simulink model "LeuchtenBox"  (R2017b)
settings: Solver=FixedStepAuto  StartTime=0.0  StopTime=10.0  RelTol=1e-3
PreLoadFcn:
  | waijung.modelPreload; % Required for working with Waijung Blockset. Do not remove.
undefined symbols (not defined in the file): HSEOSC, Link, LQFP100, m, n, ST, STM32F407VG
libraries: simulink x36, stm32f4_canbus_lib x10, stm32f4_io_lib x8, quarc_library x1, stm32f4_device_config_lib x1
CloseFcn:
  | waijung.modelClose; % Required for working with Waijung Blockset. Do not remove.
settings Model: Creator=labuser  LastModifiedBy=marti
settings OptimizationCC: DefaultParameterBehavior=Inlined  PassReuseOutputArgsAs=Individual arguments
settings DebuggingCC: ParameterTunabilityLossMsg=error
settings HardwareCC: ProdBitPerPointer=32  ProdBitPerSizeT=32  ProdBitPerPtrDiffT=32  ProdLargestAtomicFloat=None  ProdIntDivRoundTo=Undefined  ProdWordSize=32  ProdHWDeviceType=ARM Compatible->Cortex - M4  TargetEndianess=LittleEndian  TargetHWDeviceType=ARM Compatible->Cortex - M4
settings SFSimCC: MATLABDynamicMemAlloc=off
settings RTWCC: SystemTargetFile=stm32f4.tlc  GenerateMakefile=off  TemplateMakefile=ert_default_tmf  Description=STM32F4 Target  GenerateReport=on  IncludeHyperlinkInReport=on  LaunchReport=on  GenerateTraceInfo=on  GenerateTraceReport=on  GenerateTraceReportSl=on  GenerateTraceReportSf=on  GenerateTraceReportEml=on
settings CodeAppCC: ForceParamTrailComments=on  IgnoreCustomStorageClasses=off  OperatorAnnotations=on  SimulinkDataObjDesc=on  SFDataObjDesc=on  InsertBlockDesc=on
settings STFCustomTargetCC: TargetLangStandard=C99 (ISO)  MultiwordLength=256  ModelReferenceCompliant=off  CombineOutputUpdateFcns=on  ERTCustomFileBanners=on  SupportContinuousTime=off  SupportNonInlinedSFcns=off  RemoveResetFunc=on  MATLABClassNameForMDSCustomization=Simulink.SoftwareTarget.ERTCustomization  GRTInterface=off  SystemTargetFile=stm32f4.tlc
settings ERTTargetCC: TargetLangStandard=C99 (ISO)  ModelReferenceCompliant=off  ParMdlRefBuildCompliant=off  CompOptLevelCompliant=off  ConcurrentExecutionCompliant=off  ModelStepFunctionPrototypeControlCompliant=off  CPPClassGenCompliant=off  UseToolchainInfoCompliant=off  InlinedParameterPlacement=NonHierarchical  ERTSrcFileBannerTemplate=stm32f4_code_template.cgt  ERTHdrFileBannerTemplate=stm32f4_code_template.cgt  ERTDataSrcFileTemplate=stm32f4_code_template.cgt  ERTDataHdrFileTemplate=stm32f4_code_template.cgt  ERTCustomFileTemplate=stm32f4_file_process.tlc

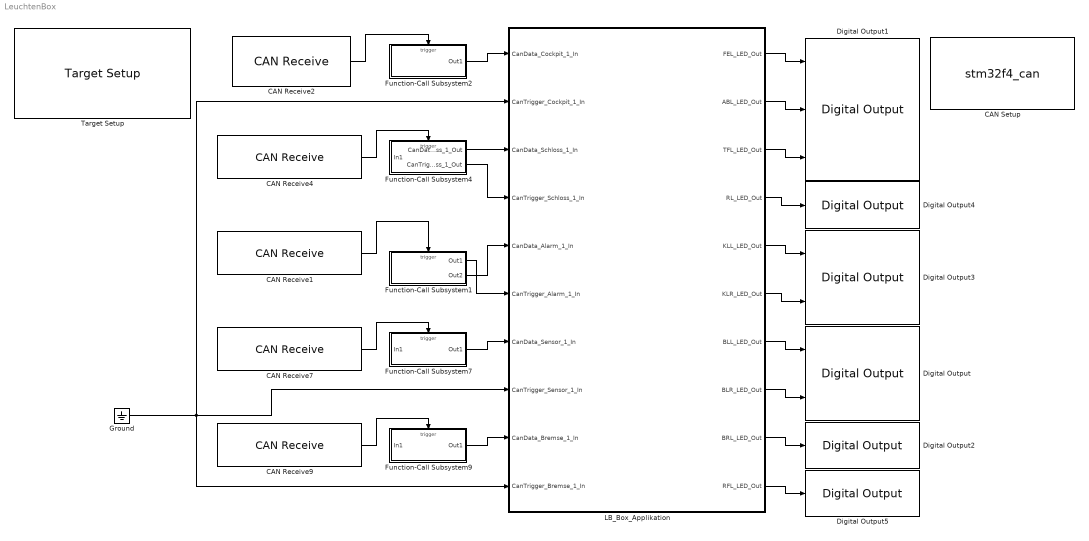
== system LeuchtenBox ==
  CAN Receive1 : stm32f4_canbus_lib/CAN Receive  conf=Rx  canmodule=1  idtype=Standard  filtertype=Specific  id=20  idmask=0  enableisr=on  usedlc=off  datatype=single  data0type=uint32  data1type=uint32  data2type=Not used  data3type=Not used  data4type=Not used  data5type=Not used  data6type=Not used  data7type=Not used  buffersize=8  sampletime=-1  sampletimestr=-1  blockid=CANReceive1  inputarray=[]  inputlabelarray={}  outputarray=[7]  outputlabelarray={'Call ISR' }  compat=0  confstr="[\"Standard\",\"Specific\",\"20\",\"0\",\"off\",\"uint32\",\"uint32\",\"Not used\",\"Not used\",\"Not used\",\"Not used\",\"Not used\",\"Not used\",\"8\",\"280\",\"0\",\"FFE0\",\"4\"]"
      settings: SourceProductName=Waijung Blockset
  CAN Receive2 : stm32f4_canbus_lib/CAN Receive  conf=Rx  canmodule=1  idtype=Standard  filtertype=Specific  id=14  idmask=0  enableisr=on  usedlc=off  datatype=single  data0type=uint32  data1type=uint32  data2type=Not used  data3type=Not used  data4type=Not used  data5type=Not used  data6type=Not used  data7type=Not used  buffersize=8  sampletime=-1  sampletimestr=-1  blockid=CANReceive2  inputarray=[]  inputlabelarray={}  outputarray=[7]  outputlabelarray={'Call ISR' }  compat=0  confstr="[\"Standard\",\"Specific\",\"14\",\"0\",\"off\",\"uint32\",\"uint32\",\"Not used\",\"Not used\",\"Not used\",\"Not used\",\"Not used\",\"Not used\",\"8\",\"1C0\",\"0\",\"FFE0\",\"4\"]"
      settings: SourceProductName=Waijung Blockset
  CAN Receive4 : stm32f4_canbus_lib/CAN Receive  conf=Rx  canmodule=1  idtype=Standard  filtertype=Specific  id=25  idmask=0  enableisr=on  usedlc=off  datatype=single  data0type=uint32  data1type=uint32  data2type=Not used  data3type=Not used  data4type=Not used  data5type=Not used  data6type=Not used  data7type=Not used  buffersize=8  sampletime=-1  sampletimestr=-1  blockid=CANReceive4  inputarray=[]  inputlabelarray={}  outputarray=[7]  outputlabelarray={'Call ISR' }  compat=0  confstr="[\"Standard\",\"Specific\",\"25\",\"0\",\"off\",\"uint32\",\"uint32\",\"Not used\",\"Not used\",\"Not used\",\"Not used\",\"Not used\",\"Not used\",\"8\",\"320\",\"0\",\"FFE0\",\"4\"]"
      settings: SourceProductName=Waijung Blockset
  CAN Receive7 : stm32f4_canbus_lib/CAN Receive  conf=Rx  canmodule=1  idtype=Standard  filtertype=Specific  id=21  idmask=0  enableisr=on  usedlc=off  datatype=single  data0type=uint32  data1type=uint32  data2type=Not used  data3type=Not used  data4type=Not used  data5type=Not used  data6type=Not used  data7type=Not used  buffersize=8  sampletime=-1  sampletimestr=-1  blockid=CANReceive7  inputarray=[]  inputlabelarray={}  outputarray=[7]  outputlabelarray={'Call ISR' }  compat=0  confstr="[\"Standard\",\"Specific\",\"21\",\"0\",\"off\",\"uint32\",\"uint32\",\"Not used\",\"Not used\",\"Not used\",\"Not used\",\"Not used\",\"Not used\",\"8\",\"2A0\",\"0\",\"FFE0\",\"4\"]"
      settings: SourceProductName=Waijung Blockset
  CAN Receive9 : stm32f4_canbus_lib/CAN Receive  conf=Rx  canmodule=1  idtype=Standard  filtertype=Specific  id=10  idmask=0  enableisr=on  usedlc=off  datatype=single  data0type=uint32  data1type=uint32  data2type=Not used  data3type=Not used  data4type=Not used  data5type=Not used  data6type=Not used  data7type=Not used  buffersize=8  sampletime=-1  sampletimestr=-1  blockid=CANReceive9  inputarray=[]  inputlabelarray={}  outputarray=[7]  outputlabelarray={'Call ISR' }  compat=0  confstr="[\"Standard\",\"Specific\",\"10\",\"0\",\"off\",\"uint32\",\"uint32\",\"Not used\",\"Not used\",\"Not used\",\"Not used\",\"Not used\",\"Not used\",\"8\",\"140\",\"0\",\"FFE0\",\"4\"]"
      settings: SourceProductName=Waijung Blockset
  CAN Setup : S-Function  FunctionName=stm32f4_can  Parameters=conf,canmodule,0,inputarray,outputarray,'','',confstr,sampletime,sampletimestr,blockid  SFunctionDeploymentMode=off  EnableBusSupport=off  mask(stm32f4_can){conf=Setup, canmodule=1, advance=off, bitrate_select=125000, sjw=1tq, bs1=14tq, bs2=6tq, timingconf=Prescaler, brp=16, bitrate=125000, tq=3.8095e-07, autoretransmission=Disable, remaptxpin=D1, remaprxpin=D0, sampletime=0.01, sampletimestr=-1, blockid=CANSetup, inputarray=[], inputlabelarray={}, outputarray=[], outputlabelarray={}, compat=0, confstr=["125000","16","D","1","D","0","1tq","14tq","6tq","ENABLE"], presc=16, txportstr=D, txpinstr=1, rxportstr=D, rxpinstr=0, lastmodule=1}
      mask prompts: conf "Configuration"; canmodule "CAN Module"; advance "Advance configuration"; bitrate_select "Baud rate (bps)"; sjw "Resync Jump Width (SJW)"; bs1 "Bit segment 1 (BS1) + PROP_SEG"; bs2 "Bit segment 2 (BS2)"; timingconf "Adjust"; brp "Baud rate prescaler (BRP)"; bitrate "Baud rate (bps)"; tq "Time Quantum (Second), tq"; autoretransmission "Auto Re-transmission"; remaptxpin "CAN Tx pin"; remaprxpin "CAN Rx pin"; sampletime "Sample time (sec)"; sampletimestr "Compiled sample time (sec) in string"; inputarray "Input port"; inputlabelarray "Input port label"; outputarray "Output port"; outputlabelarray "Output port label"; compat "Compatibility (Reserved for future use)"; confstr "Configuration String"; presc "Prescale"; txportstr "Tx port string"; txpinstr "Tx pin string"; rxportstr "Rx port string"; rxpinstr "Rx pin string"; lastmodule "Last module selected"
      mask help:
      | This block setups CAN Module.
      |
      | Auto Re-transmission,
      |  - Enable: The CAN hardware will automatically retransmit the message until it has been
      | successfully transmitted according to the CAN standard.
      |  - Disable: A message will be transmitted only once, independently of the transmission result
      | (successful, error or arbitration lost).
      mask init:
      | stm32f4_can_callback('init');
      mask Help: web(fullfile(waijungdocroot,'stm32f4_can_setup.htm'), '-browser')
      mask TypeOptions conf: Setup
      mask TypeOptions canmodule: 1 | 2
      mask Callback canmodule: stm32f4_can_callback('canmodule');
      mask Callback advance: stm32f4_can_callback('advance');
      mask TypeOptions bitrate_select: 125000 | 250000 | 500000 | 1000000
      mask Callback bitrate_select: stm32f4_can_callback('bitrate_select');
      mask TypeOptions sjw: 1tq | 2tq | 3tq | 4tq
      mask TypeOptions bs1: 1tq | 2tq | 3tq | 4tq | 5tq | 6tq | 7tq | 8tq | 9tq | 10tq | 11tq | 12tq | 13tq | 14tq | 15tq | 16tq
      mask Callback bs1: stm32f4_can_callback('timingconf');
      mask TypeOptions bs2: 1tq | 2tq | 3tq | 4tq | 5tq | 6tq | 7tq | 8tq
      mask Callback bs2: stm32f4_can_callback('timingconf');
      mask TypeOptions timingconf: Prescaler | Baudrate
      mask Callback timingconf: stm32f4_can_callback('timingconf');
      mask Callback brp: stm32f4_can_callback('timingconf');
      mask Callback bitrate: stm32f4_can_callback('timingconf');
      mask TypeOptions autoretransmission: Enable | Disable
      mask TypeOptions remaptxpin: Not used | A12 | B9 | D1
      mask Callback remaptxpin: stm32f4_can_callback('remaptxpin');
      mask TypeOptions remaprxpin: Not used | A11 | B8 | D0
      mask Callback remaprxpin: stm32f4_can_callback('remaprxpin');
      mask Callback sampletime: stm32f4_can_callback('sampletime');
      mask Callback sampletimestr: stm32f4_can_callback('sampletimestr');
      mask Callback blockid: stm32f4_can_callback('blockid');
      mask Display: text(0.5, 0.5, 'CAN1_Setup\nSpeed (bps): 125000\nTx/Rx pin: D1/D0','ver','middle','hor','center');
  Digital Output : stm32f4_io_lib/Digital Output  use_bitband=on  port=C  speed=100  porttype=Push Pull  porttypestr=PP  use_pin0=on  use_pin1=on  use_pin2=off  use_pin3=off  use_pin4=off  use_pin5=off  use_pin6=off  use_pin7=off  use_pin8=off  use_pin9=off  use_pin10=off  use_pin11=off  use_pin12=off  use_pin13=off  use_pin14=off  use_pin15=off  pinstr=GPIO_Pin_0 | GPIO_Pin_1  usedpinarray="[1  1  0  0  0  0  0  0  0  0  0  0  0  0  0  0]"  bitbandingstr=|  sampletime=-1  sampletimestr=-1  blockid=DigitalOutput  enablecustomportlabel=off  globalinit=off  cinputportlabel=In1, In2  coutputportlabel=0
      | #define DigitalOutput_C0 Peripheral_BB(GPIOC->ODR, 0)  /* Output pin */
      | #define DigitalOutput_C1 Peripheral_BB(GPIOC->ODR, 1)  /* Output pin */
      settings: SourceProductName=Waijung Blockset
  Digital Output1 : stm32f4_io_lib/Digital Output  use_bitband=on  port=C  speed=100  porttype=Push Pull  porttypestr=PP  use_pin0=off  use_pin1=off  use_pin2=on  use_pin3=on  use_pin4=on  use_pin5=off  use_pin6=off  use_pin7=off  use_pin8=off  use_pin9=off  use_pin10=off  use_pin11=off  use_pin12=off  use_pin13=off  use_pin14=off  use_pin15=off  pinstr=GPIO_Pin_2 | GPIO_Pin_3 | GPIO_Pin_4  usedpinarray="[0  0  1  1  1  0  0  0  0  0  0  0  0  0  0  0]"  bitbandingstr=|  sampletime=-1  sampletimestr=-1  blockid=DigitalOutput1  enablecustomportlabel=off  globalinit=off  cinputportlabel=In1, In2  coutputportlabel=0
      | #define DigitalOutput1_C2 Peripheral_BB(GPIOC->ODR, 2)  /* Output pin */
      | #define DigitalOutput1_C3 Peripheral_BB(GPIOC->ODR, 3)  /* Output pin */
      | #define DigitalOutput1_C4 Peripheral_BB(GPIOC->ODR, 4)  /* Output pin */
      settings: SourceProductName=Waijung Blockset
  Digital Output2 : stm32f4_io_lib/Digital Output  use_bitband=on  port=C  speed=100  porttype=Push Pull  porttypestr=PP  use_pin0=off  use_pin1=off  use_pin2=off  use_pin3=off  use_pin4=off  use_pin5=on  use_pin6=off  use_pin7=off  use_pin8=off  use_pin9=off  use_pin10=off  use_pin11=off  use_pin12=off  use_pin13=off  use_pin14=off  use_pin15=off  pinstr=GPIO_Pin_5  usedpinarray="[0  0  0  0  0  1  0  0  0  0  0  0  0  0  0  0]"  bitbandingstr="#define DigitalOutput2_C5 Peripheral_BB(GPIOC->ODR, 5)  /* Output pin */"  sampletime=-1  sampletimestr=-1  blockid=DigitalOutput2  enablecustomportlabel=off  globalinit=off  cinputportlabel=In1, In2  coutputportlabel=0
      settings: SourceProductName=Waijung Blockset
  Digital Output3 : stm32f4_io_lib/Digital Output  use_bitband=on  port=C  speed=100  porttype=Push Pull  porttypestr=PP  use_pin0=off  use_pin1=off  use_pin2=off  use_pin3=off  use_pin4=off  use_pin5=off  use_pin6=off  use_pin7=on  use_pin8=off  use_pin9=on  use_pin10=off  use_pin11=off  use_pin12=off  use_pin13=off  use_pin14=off  use_pin15=off  pinstr=GPIO_Pin_7 | GPIO_Pin_9  usedpinarray="[0  0  0  0  0  0  0  1  0  1  0  0  0  0  0  0]"  bitbandingstr=|  sampletime=-1  sampletimestr=-1  blockid=DigitalOutput3  enablecustomportlabel=off  globalinit=off  cinputportlabel=In1, In2  coutputportlabel=0
      | #define DigitalOutput3_C7 Peripheral_BB(GPIOC->ODR, 7)  /* Output pin */
      | #define DigitalOutput3_C9 Peripheral_BB(GPIOC->ODR, 9)  /* Output pin */
      settings: SourceProductName=Waijung Blockset
  Digital Output4 : stm32f4_io_lib/Digital Output  use_bitband=on  port=C  speed=100  porttype=Push Pull  porttypestr=PP  use_pin0=off  use_pin1=off  use_pin2=off  use_pin3=off  use_pin4=off  use_pin5=off  use_pin6=off  use_pin7=off  use_pin8=on  use_pin9=off  use_pin10=off  use_pin11=off  use_pin12=off  use_pin13=off  use_pin14=off  use_pin15=off  pinstr=GPIO_Pin_8  usedpinarray="[0  0  0  0  0  0  0  0  1  0  0  0  0  0  0  0]"  bitbandingstr="#define DigitalOutput4_C8 Peripheral_BB(GPIOC->ODR, 8)  /* Output pin */"  sampletime=-1  sampletimestr=-1  blockid=DigitalOutput4  enablecustomportlabel=off  globalinit=off  cinputportlabel=In1, In2  coutputportlabel=0
      settings: SourceProductName=Waijung Blockset
  Digital Output5 : stm32f4_io_lib/Digital Output  use_bitband=on  port=C  speed=100  porttype=Push Pull  porttypestr=PP  use_pin0=off  use_pin1=off  use_pin2=off  use_pin3=off  use_pin4=off  use_pin5=off  use_pin6=on  use_pin7=off  use_pin8=off  use_pin9=off  use_pin10=off  use_pin11=off  use_pin12=off  use_pin13=off  use_pin14=off  use_pin15=off  pinstr=GPIO_Pin_6  usedpinarray="[0  0  0  0  0  0  1  0  0  0  0  0  0  0  0  0]"  bitbandingstr="#define DigitalOutput5_C6 Peripheral_BB(GPIOC->ODR, 6)  /* Output pin */"  sampletime=-1  sampletimestr=-1  blockid=DigitalOutput5  enablecustomportlabel=off  globalinit=off  cinputportlabel=In1, In2  coutputportlabel=0
      settings: SourceProductName=Waijung Blockset
  Function-Call Subsystem1 : Subsystem  TreatAsAtomicUnit=on
  Function-Call Subsystem2 : Subsystem  TreatAsAtomicUnit=on
  Function-Call Subsystem4 : Subsystem  TreatAsAtomicUnit=on
  Function-Call Subsystem7 : Subsystem  TreatAsAtomicUnit=on
  Function-Call Subsystem9 : Subsystem  TreatAsAtomicUnit=on
  Ground : Ground
  LB_Box_Applikation : Subsystem
  Target Setup : stm32f4_device_config_lib/Target Setup  Priority=100  compiler=GNU ARM  previous_compiler=GNU ARM  mcu=STM32F407VG (LQFP100)  mcustr=STM32F407VG  clockconfig=HSEOSC-8MHz  system_stm32f4xx_c_path=C:\waijung17_03a\targets\stm32f4_target\stm32f4\utils\system_stm32f4xx_default\STM32F40_41xxx\hseosc8mhz  showmemoryconfiguration=off  stacksize=0x2000  heapsize=0x2000  enableautocompiledownload=on  fullchiperase=off  programmerinterface=ST-Link  editctrlstr=on  compilercontrolstr=$(patsubst %, -I%, .) -mcpu=cortex-m4 -mthumb -mthumb-interwork -mfloat-abi=hard -mfpu=fpv4-sp-d16 -ffast-math -Wall -Wextra -Ofast  assemblercontrolstr=$(patsubst %, -I%, .) -mcpu=cortex-m4 -mthumb -mthumb-interwork -mfloat-abi=hard -mfpu=fpv4-sp-d16 -ffast-math -Wall -Wextra -Ofast -Wa,-amhls=$(<:.s=.lst) -D__STACK_SIZE=$(STACK_SIZE) -D__HEAP_SIZE=$(HEAP_SIZE)  linkercontrolstr=-T$(LD_SCRIPT) -g -Wl,-Map=$(MAP),--cref,--no-warn-mismatch -mcpu=cortex-m4 -mthumb -mthumb-interwork -mfloat-abi=hard -mfpu=fpv4-sp-d16 -specs=nosys.specs  runafterdownload=on  execprofile=None  profileruart=3  profilerbaud=500000  profilertxpin=D8  profilerinitstr=0.01,168000000,1680000,500000,0  manualsetsampletime=off  sampletime=0.01  blockid=TargetSetup  systickreloadvalue=1680000  hseval=8000000  lastprofileruart=3  hclk=168000000  flashorigin=0x8000000  flashlength=1024k  ramorigin=0x20000000  ramlength=128k  useextram=off
      settings: SourceProductName=Waijung Blockset
  wires:
  LB_Box_Applikation/7(BLL_LED_Out) -> Digital Output/1
  LB_Box_Applikation/8(BLR_LED_Out) -> Digital Output/2
  LB_Box_Applikation/1(FEL_LED_Out) -> Digital Output1/1
  LB_Box_Applikation/2(ABL_LED_Out) -> Digital Output1/2
  LB_Box_Applikation/3(TFL_LED_Out) -> Digital Output1/3
  LB_Box_Applikation/9(BRL_LED_Out) -> Digital Output2/1
  LB_Box_Applikation/5(KLL_LED_Out) -> Digital Output3/1
  LB_Box_Applikation/6(KLR_LED_Out) -> Digital Output3/2
  LB_Box_Applikation/4(RL_LED_Out) -> Digital Output4/1
  LB_Box_Applikation/10(RFL_LED_Out) -> Digital Output5/1
  CAN Receive2/1 -> Function-Call Subsystem2/Trigger
  Function-Call Subsystem2/1(Out1) -> LB_Box_Applikation/1(CanData_Cockpit_1_In)
  Function-Call Subsystem4/1(CanData_Schloss_1_Out) -> LB_Box_Applikation/3(CanData_Schloss_1_In)
  CAN Receive4/1 -> Function-Call Subsystem4/Trigger
  CAN Receive7/1 -> Function-Call Subsystem7/Trigger
  CAN Receive1/1 -> Function-Call Subsystem1/Trigger
  Function-Call Subsystem7/1(Out1) -> LB_Box_Applikation/7(CanData_Sensor_1_In)
  Function-Call Subsystem9/1(Out1) -> LB_Box_Applikation/9(CanData_Bremse_1_In)
  CAN Receive9/1 -> Function-Call Subsystem9/Trigger
  Ground/1 -> LB_Box_Applikation/8(CanTrigger_Sensor_1_In), LB_Box_Applikation/2(CanTrigger_Cockpit_1_In), LB_Box_Applikation/10(CanTrigger_Bremse_1_In)
  Function-Call Subsystem1/2(Out2) -> LB_Box_Applikation/5(CanData_Alarm_1_In)
  Function-Call Subsystem1/1(Out1) -> LB_Box_Applikation/6(CanTrigger_Alarm_1_In)
  Function-Call Subsystem4/2(CanTrigger_Schloss_1_Out) -> LB_Box_Applikation/4(CanTrigger_Schloss_1_In)

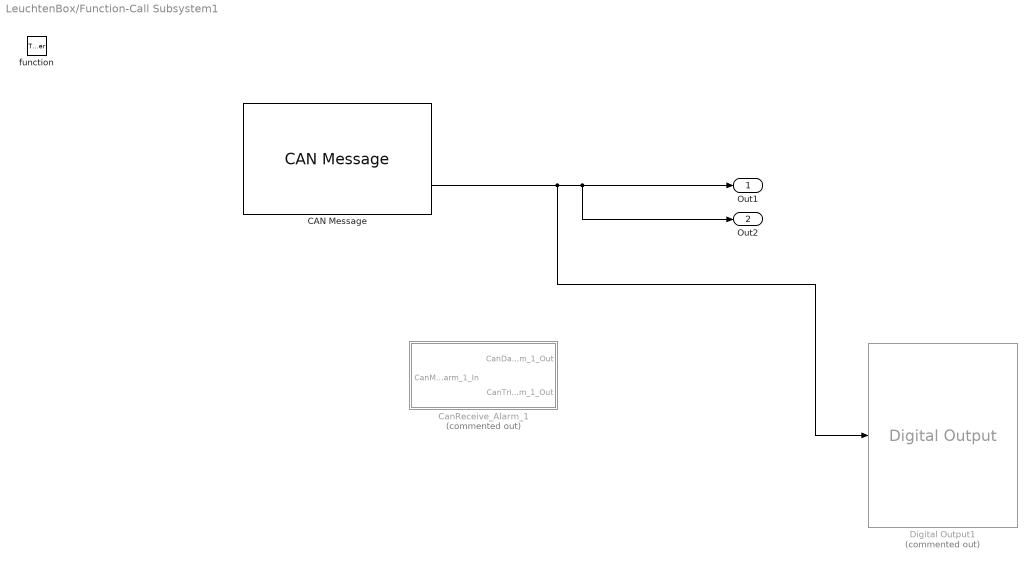
== system LeuchtenBox/Function-Call Subsystem1 ==
  function : TriggerPort  TriggerType=function-call  VariantControl=Variant
  CAN Message : stm32f4_canbus_lib/CAN Message  conf=Msg  canmodule=1  usedlc=off  datatype=double  data0type=uint8  data1type=Not used  data2type=Not used  data3type=Not used  data4type=Not used  data5type=Not used  data6type=Not used  data7type=Not used  sampletime=-1  sampletimestr=-1  blockid=FunctionCallSubsystem1CANMessage  inputarray=[]  inputlabelarray={}  outputarray=[ 7, 3]  outputlabelarray={'ID', 'D0 (uint8)' }  compat=0  confstr="[\"off\",\"uint8\",\"Not used\",\"Not used\",\"Not used\",\"Not used\",\"Not used\",\"Not used\",\"Not used\"]"
      settings: SourceProductName=Waijung Blockset
  CanReceive_Alarm_1 : Subsystem  Commented=on
  Digital Output1 : stm32f4_io_lib/Digital Output  Commented=on  use_bitband=on  port=C  speed=100  porttype=Push Pull  porttypestr=PP  use_pin0=off  use_pin1=off  use_pin2=off  use_pin3=on  use_pin4=off  use_pin5=off  use_pin6=off  use_pin7=off  use_pin8=off  use_pin9=off  use_pin10=off  use_pin11=off  use_pin12=off  use_pin13=off  use_pin14=off  use_pin15=off  pinstr=GPIO_Pin_3  usedpinarray="[0  0  0  1  0  0  0  0  0  0  0  0  0  0  0  0]"  bitbandingstr="#define FunctionCallSubsystem1DigitalOutput1_C3 Peripheral_BB(GPIOC->ODR, 3)  /* Output pin */"  sampletime=-1  sampletimestr=-1  blockid=FunctionCallSubsystem1DigitalOutput1  enablecustomportlabel=off  globalinit=off  cinputportlabel=In1, In2  coutputportlabel=0
      settings: SourceProductName=Waijung Blockset
  Out1 : Outport
  Out2 : Outport  Port=2
  wires:
  CAN Message/2 -> Digital Output1/1, Out2/1, Out1/1

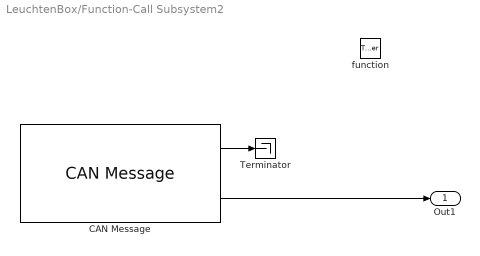
== system LeuchtenBox/Function-Call Subsystem2 ==
  function : TriggerPort  TriggerType=function-call  VariantControl=Variant
  CAN Message : stm32f4_canbus_lib/CAN Message  conf=Msg  canmodule=1  usedlc=off  datatype=double  data0type=uint16  data1type=Not used  data2type=Not used  data3type=Not used  data4type=Not used  data5type=Not used  data6type=Not used  data7type=Not used  sampletime=-1  sampletimestr=-1  blockid=FunctionCallSubsystem2CANMessage  inputarray=[]  inputlabelarray={}  outputarray=[ 7, 5]  outputlabelarray={'ID', 'D0 (uint16)' }  compat=0  confstr="[\"off\",\"uint16\",\"Not used\",\"Not used\",\"Not used\",\"Not used\",\"Not used\",\"Not used\",\"Not used\"]"
      settings: SourceProductName=Waijung Blockset
  Terminator : Terminator
  Out1 : Outport
  wires:
  CAN Message/1 -> Terminator/1
  CAN Message/2 -> Out1/1

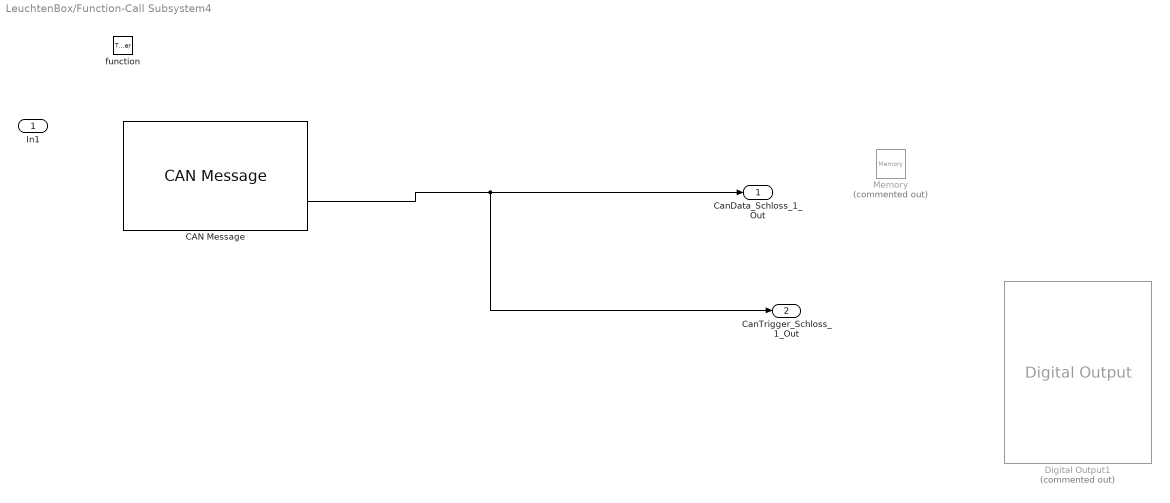
== system LeuchtenBox/Function-Call Subsystem4 ==
  In1 : Inport
  function : TriggerPort  TriggerType=function-call  VariantControl=Variant
  CAN Message : stm32f4_canbus_lib/CAN Message  conf=Msg  canmodule=1  usedlc=off  datatype=double  data0type=uint8  data1type=Not used  data2type=Not used  data3type=Not used  data4type=Not used  data5type=Not used  data6type=Not used  data7type=Not used  sampletime=-1  sampletimestr=-1  blockid=FunctionCallSubsystem4CANMessage  inputarray=[]  inputlabelarray={}  outputarray=[ 7, 3]  outputlabelarray={'ID', 'D0 (uint8)' }  compat=0  confstr="[\"off\",\"uint8\",\"Not used\",\"Not used\",\"Not used\",\"Not used\",\"Not used\",\"Not used\",\"Not used\"]"
      settings: SourceProductName=Waijung Blockset
  Digital Output1 : stm32f4_io_lib/Digital Output  Commented=on  use_bitband=on  port=C  speed=100  porttype=Push Pull  porttypestr=PP  use_pin0=off  use_pin1=off  use_pin2=off  use_pin3=on  use_pin4=off  use_pin5=off  use_pin6=off  use_pin7=off  use_pin8=off  use_pin9=off  use_pin10=off  use_pin11=off  use_pin12=off  use_pin13=off  use_pin14=off  use_pin15=off  pinstr=GPIO_Pin_3  usedpinarray="[0  0  0  1  0  0  0  0  0  0  0  0  0  0  0  0]"  bitbandingstr="#define FunctionCallSubsystem4DigitalOutput1_C3 Peripheral_BB(GPIOC->ODR, 3)  /* Output pin */"  sampletime=-1  sampletimestr=-1  blockid=FunctionCallSubsystem4DigitalOutput1  enablecustomportlabel=off  globalinit=off  cinputportlabel=In1, In2  coutputportlabel=0
      settings: SourceProductName=Waijung Blockset
  Memory : quarc_library/Discrete/Memory  Commented=on  initial_condition=0  sample_time=-1
      settings: SourceProductName=QUARC Targets
  CanData_Schloss_1_Out : Outport
  CanTrigger_Schloss_1_Out : Outport  Port=2
  wires:
  CAN Message/2 -> CanTrigger_Schloss_1_Out/1, CanData_Schloss_1_Out/1

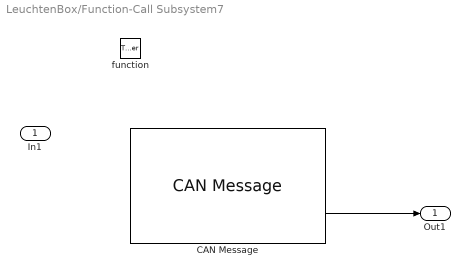
== system LeuchtenBox/Function-Call Subsystem7 ==
  In1 : Inport
  function : TriggerPort  TriggerType=function-call  VariantControl=Variant
  CAN Message : stm32f4_canbus_lib/CAN Message  conf=Msg  canmodule=1  usedlc=off  datatype=double  data0type=uint16  data1type=Not used  data2type=Not used  data3type=Not used  data4type=Not used  data5type=Not used  data6type=Not used  data7type=Not used  sampletime=-1  sampletimestr=-1  blockid=FunctionCallSubsystem7CANMessage  inputarray=[]  inputlabelarray={}  outputarray=[ 7, 5]  outputlabelarray={'ID', 'D0 (uint16)' }  compat=0  confstr="[\"off\",\"uint16\",\"Not used\",\"Not used\",\"Not used\",\"Not used\",\"Not used\",\"Not used\",\"Not used\"]"
      settings: SourceProductName=Waijung Blockset
  Out1 : Outport
  wires:
  CAN Message/2 -> Out1/1

== system LeuchtenBox/Function-Call Subsystem9 ==
  In1 : Inport
  function : TriggerPort  TriggerType=function-call  VariantControl=Variant
  CAN Message : stm32f4_canbus_lib/CAN Message  conf=Msg  canmodule=1  usedlc=off  datatype=double  data0type=uint8  data1type=Not used  data2type=Not used  data3type=Not used  data4type=Not used  data5type=Not used  data6type=Not used  data7type=Not used  sampletime=-1  sampletimestr=-1  blockid=FunctionCallSubsystem9CANMessage  inputarray=[]  inputlabelarray={}  outputarray=[ 7, 3]  outputlabelarray={'ID', 'D0 (uint8)' }  compat=0  confstr="[\"off\",\"uint8\",\"Not used\",\"Not used\",\"Not used\",\"Not used\",\"Not used\",\"Not used\",\"Not used\"]"
      settings: SourceProductName=Waijung Blockset
  Out1 : Outport
  wires:
  CAN Message/2 -> Out1/1

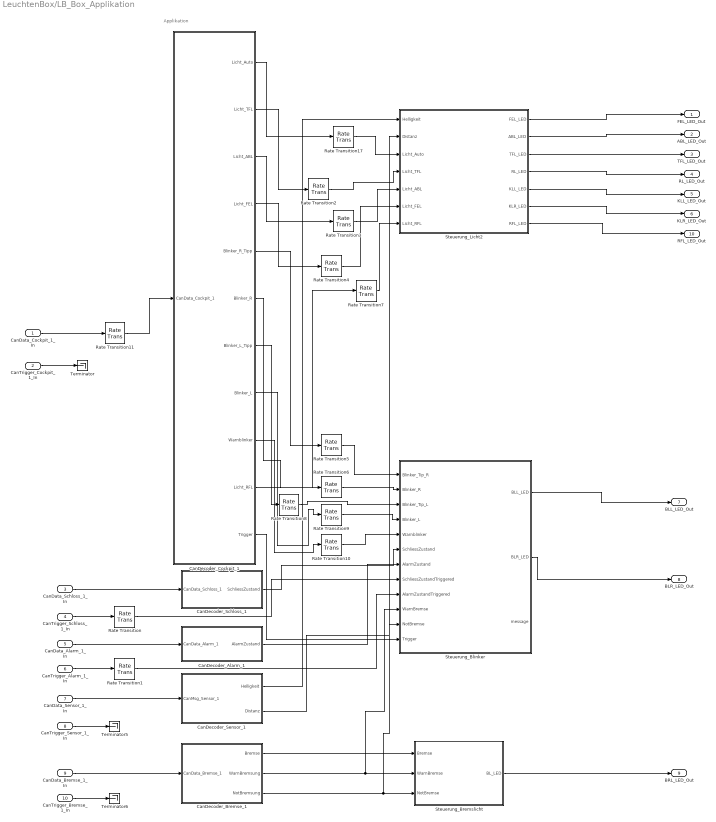
== system LeuchtenBox/LB_Box_Applikation ==
  note: Applikation
  CanData_Cockpit_1_In : Inport
  CanTrigger_Cockpit_1_In : Inport  Port=2
  CanData_Schloss_1_In : Inport  Port=3
  CanTrigger_Schloss_1_In : Inport  Port=4
  CanData_Alarm_1_In : Inport  Port=5
  CanTrigger_Alarm_1_In : Inport  Port=6
  CanData_Sensor_1_In : Inport  Port=7
  CanTrigger_Sensor_1_In : Inport  Port=8
  CanData_Bremse_1_In : Inport  Port=9
  CanTrigger_Bremse_1_In : Inport  Port=10
  CanDecoder_Alarm_1 : Subsystem
  CanDecoder_Bremse_1 : Subsystem
  CanDecoder_Cockpit_1 : Subsystem
  CanDecoder_Schloss_1 : Subsystem
  CanDecoder_Sensor_1 : Subsystem
  Rate Transition{,1..11,17} (13 alike) : RateTransition  Deterministic=off
  Steuerung_Blinker : Stateflow chart  TreatAsAtomicUnit=on
  Steuerung_Bremslicht : Stateflow chart  TreatAsAtomicUnit=on
  Steuerung_Licht2 : Stateflow chart  TreatAsAtomicUnit=on
  Terminator : Terminator
  Terminator5 : Terminator
  Terminator6 : Terminator
  FEL_LED_Out : Outport
  ABL_LED_Out : Outport  Port=2
  TFL_LED_Out : Outport  Port=3
  RL_LED_Out : Outport  Port=4
  KLL_LED_Out : Outport  Port=5
  KLR_LED_Out : Outport  Port=6
  BLL_LED_Out : Outport  Port=7
  BLR_LED_Out : Outport  Port=8
  BRL_LED_Out : Outport  Port=9
  RFL_LED_Out : Outport  Port=10
  wires:
  Steuerung_Blinker/2(BLR_LED) -> BLR_LED_Out/1
  Steuerung_Licht2/2(ABL_LED) -> ABL_LED_Out/1
  Steuerung_Blinker/1(BLL_LED) -> BLL_LED_Out/1
  CanDecoder_Bremse_1/2(WarnBremsung) -> Steuerung_Blinker/10(WarnBremse), Steuerung_Bremslicht/2(WarnBremse)
  CanDecoder_Cockpit_1/3(Licht_ABL) -> Rate Transition3/1
  CanDecoder_Sensor_1/1(Helligkeit) -> Steuerung_Licht2/1(Helligkeit)
  CanDecoder_Schloss_1/1(SchliessZustand) -> Steuerung_Blinker/6(SchliessZustand)
  CanDecoder_Alarm_1/1(AlarmZustand) -> Steuerung_Blinker/7(AlarmZustand)
  CanDecoder_Cockpit_1/2(Licht_TFL) -> Rate Transition2/1
  CanData_Sensor_1_In/1 -> CanDecoder_Sensor_1/1(CanMsg_Sensor_1)
  CanData_Cockpit_1_In/1 -> Rate Transition11/1
  CanData_Schloss_1_In/1 -> CanDecoder_Schloss_1/1(CanData_Schloss_1)
  CanData_Alarm_1_In/1 -> CanDecoder_Alarm_1/1(CanData_Alarm_1)
  CanData_Bremse_1_In/1 -> CanDecoder_Bremse_1/1(CanData_Bremse_1)
  CanTrigger_Cockpit_1_In/1 -> Terminator/1
  CanTrigger_Schloss_1_In/1 -> Rate Transition/1
  CanTrigger_Alarm_1_In/1 -> Rate Transition1/1
  CanTrigger_Sensor_1_In/1 -> Terminator5/1
  CanTrigger_Bremse_1_In/1 -> Terminator6/1
  Steuerung_Licht2/1(FEL_LED) -> FEL_LED_Out/1
  Steuerung_Licht2/3(TFL_LED) -> TFL_LED_Out/1
  CanDecoder_Bremse_1/3(NotBremsung) -> Steuerung_Blinker/11(NotBremse), Steuerung_Bremslicht/3(NotBremse)
  Steuerung_Bremslicht/1(BL_LED) -> BRL_LED_Out/1
  CanDecoder_Bremse_1/1(Bremse) -> Steuerung_Bremslicht/1(Bremse)
  CanDecoder_Cockpit_1/1(Licht_Auto) -> Rate Transition17/1
  Steuerung_Licht2/4(RL_LED) -> RL_LED_Out/1
  Steuerung_Licht2/5(KLL_LED) -> KLL_LED_Out/1
  Steuerung_Licht2/6(KLR_LED) -> KLR_LED_Out/1
  CanDecoder_Sensor_1/2(Distanz) -> Steuerung_Licht2/2(Distanz)
  CanDecoder_Cockpit_1/4(Licht_FEL) -> Rate Transition4/1
  CanDecoder_Cockpit_1/10(Licht_RFL) -> Rate Transition7/1
  CanDecoder_Cockpit_1/5(Blinker_R_Tipp) -> Rate Transition5/1
  CanDecoder_Cockpit_1/6(Blinker_R) -> Rate Transition6/1
  CanDecoder_Cockpit_1/7(Blinker_L_Tipp) -> Rate Transition8/1
  CanDecoder_Cockpit_1/8(Blinker_L) -> Rate Transition9/1
  CanDecoder_Cockpit_1/9(Warnblinker) -> Rate Transition10/1
  Steuerung_Licht2/7(RFL_LED) -> RFL_LED_Out/1
  Rate Transition/1 -> Steuerung_Blinker/8(SchliessZustandTriggered)
  Rate Transition1/1 -> Steuerung_Blinker/9(AlarmZustandTriggered)
  Rate Transition17/1 -> Steuerung_Licht2/3(Licht_Auto)
  Rate Transition2/1 -> Steuerung_Licht2/4(Licht_TFL)
  Rate Transition3/1 -> Steuerung_Licht2/5(Licht_ABL)
  Rate Transition4/1 -> Steuerung_Licht2/6(Licht_FEL)
  Rate Transition5/1 -> Steuerung_Blinker/1(Blinker_Tip_R)
  Rate Transition6/1 -> Steuerung_Blinker/2(Blinker_R)
  Rate Transition7/1 -> Steuerung_Licht2/7(Licht_RFL)
  Rate Transition8/1 -> Steuerung_Blinker/3(Blinker_Tip_L)
  Rate Transition9/1 -> Steuerung_Blinker/4(Blinker_L)
  Rate Transition10/1 -> Steuerung_Blinker/5(Warnblinker)
  Rate Transition11/1 -> CanDecoder_Cockpit_1/1(CanData_Cockpit_1)
  CanDecoder_Cockpit_1/11(Trigger) -> Steuerung_Blinker/12(Trigger)

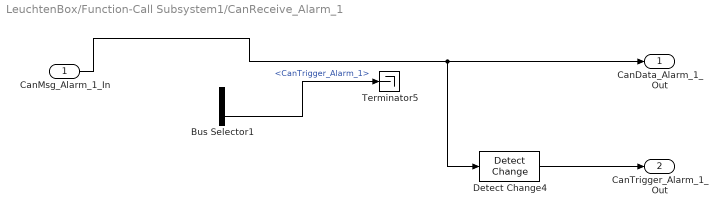
== system LeuchtenBox/Function-Call Subsystem1/CanReceive_Alarm_1 ==
  CanMsg_Alarm_1_In : Inport
  Bus Selector1 : BusSelector  OutputSignals=CanData_Alarm_1,CanTrigger_Alarm_1
  Detect Change4 : simulink/Logic and Bit Operations/Detect Change  vinit=0  OutDataTypeStr=boolean
  Terminator5 : Terminator
  CanData_Alarm_1_Out : Outport
  CanTrigger_Alarm_1_Out : Outport  Port=2
  wires:
  CanMsg_Alarm_1_In/1 -> Detect Change4/1, CanData_Alarm_1_Out/1
  Bus Selector1/2 -> Terminator5/1  "<CanTrigger_Alarm_1>"
  Detect Change4/1 -> CanTrigger_Alarm_1_Out/1

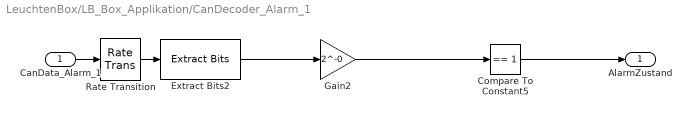
== system LeuchtenBox/LB_Box_Applikation/CanDecoder_Alarm_1 ==
  CanData_Alarm_1 : Inport
  Compare To Constant5 : simulink/Logic and Bit Operations/Compare To Constant  relop===  const=1  OutDataTypeStr=boolean
  Extract Bits2 : simulink/Logic and Bit Operations/Extract Bits  bitsToExtract=Range of bits  numBits=8  bitIdxRange=0  outScalingMode=Preserve fixed-point scaling
  Gain2 : Gain  Gain=2^-0
  Rate Transition : RateTransition  Deterministic=off
  AlarmZustand : Outport
  wires:
  Gain2/1 -> Compare To Constant5/1
  Extract Bits2/1 -> Gain2/1
  CanData_Alarm_1/1 -> Rate Transition/1
  Compare To Constant5/1 -> AlarmZustand/1
  Rate Transition/1 -> Extract Bits2/1

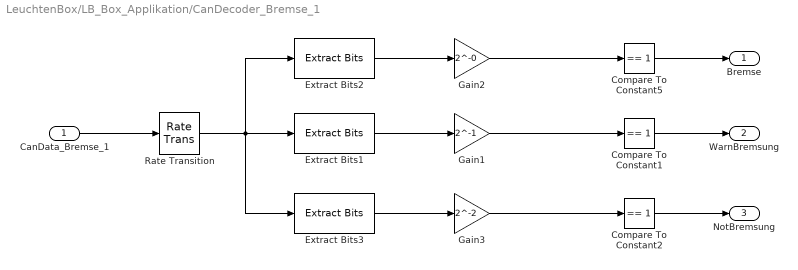
== system LeuchtenBox/LB_Box_Applikation/CanDecoder_Bremse_1 ==
  CanData_Bremse_1 : Inport
  Compare To Constant1 : simulink/Logic and Bit Operations/Compare To Constant  relop===  const=1  OutDataTypeStr=boolean
  Compare To Constant2 : simulink/Logic and Bit Operations/Compare To Constant  relop===  const=1  OutDataTypeStr=boolean
  Compare To Constant5 : simulink/Logic and Bit Operations/Compare To Constant  relop===  const=1  OutDataTypeStr=boolean
  Extract Bits1 : simulink/Logic and Bit Operations/Extract Bits  bitsToExtract=Range of bits  numBits=8  bitIdxRange=1  outScalingMode=Preserve fixed-point scaling
  Extract Bits2 : simulink/Logic and Bit Operations/Extract Bits  bitsToExtract=Range of bits  numBits=8  bitIdxRange=0  outScalingMode=Preserve fixed-point scaling
  Extract Bits3 : simulink/Logic and Bit Operations/Extract Bits  bitsToExtract=Range of bits  numBits=8  bitIdxRange=2  outScalingMode=Preserve fixed-point scaling
  Gain1 : Gain  Gain=2^-1
  Gain2 : Gain  Gain=2^-0
  Gain3 : Gain  Gain=2^-2
  Rate Transition : RateTransition  Deterministic=off
  Bremse : Outport
  WarnBremsung : Outport  Port=2
  NotBremsung : Outport  Port=3
  wires:
  CanData_Bremse_1/1 -> Rate Transition/1
  Gain2/1 -> Compare To Constant5/1
  Extract Bits2/1 -> Gain2/1
  Gain1/1 -> Compare To Constant1/1
  Extract Bits1/1 -> Gain1/1
  Compare To Constant1/1 -> WarnBremsung/1
  Compare To Constant5/1 -> Bremse/1
  Gain3/1 -> Compare To Constant2/1
  Extract Bits3/1 -> Gain3/1
  Compare To Constant2/1 -> NotBremsung/1
  Rate Transition/1 -> Extract Bits2/1, Extract Bits1/1, Extract Bits3/1

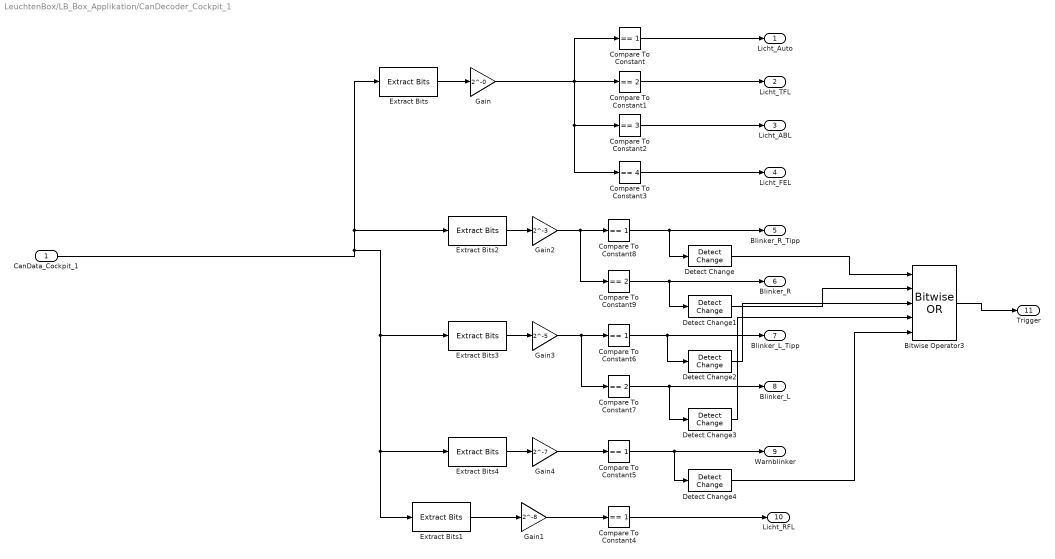
== system LeuchtenBox/LB_Box_Applikation/CanDecoder_Cockpit_1 ==
  CanData_Cockpit_1 : Inport
  Bitwise Operator3 : simulink/Logic and Bit Operations/Bitwise Operator  logicop=OR  UseBitMask=off  NumInputPorts=5  BitMask=bin2dec('11011001')  BitMaskRealWorld=Stored Integer
  Compare To Constant{,4..6,8} (5 alike) : simulink/Logic and Bit Operations/Compare To Constant  relop===  const=1  OutDataTypeStr=boolean
  Compare To Constant1 : simulink/Logic and Bit Operations/Compare To Constant  relop===  const=2  OutDataTypeStr=boolean
  Compare To Constant2 : simulink/Logic and Bit Operations/Compare To Constant  relop===  const=3  OutDataTypeStr=boolean
  Compare To Constant3 : simulink/Logic and Bit Operations/Compare To Constant  relop===  const=4  OutDataTypeStr=boolean
  Compare To Constant7 : simulink/Logic and Bit Operations/Compare To Constant  relop===  const=2  OutDataTypeStr=boolean
  Compare To Constant9 : simulink/Logic and Bit Operations/Compare To Constant  relop===  const=2  OutDataTypeStr=boolean
  Detect Change{,1..4} (5 alike) : simulink/Logic and Bit Operations/Detect Change  vinit=0  OutDataTypeStr=boolean
  Extract Bits : simulink/Logic and Bit Operations/Extract Bits  bitsToExtract=Range of bits  numBits=8  bitIdxRange=[0 2]  outScalingMode=Preserve fixed-point scaling
      settings: SourceProductName=Simulink
  Extract Bits1 : simulink/Logic and Bit Operations/Extract Bits  bitsToExtract=Range of bits  numBits=8  bitIdxRange=8  outScalingMode=Preserve fixed-point scaling
      settings: SourceProductName=Simulink
  Extract Bits2 : simulink/Logic and Bit Operations/Extract Bits  bitsToExtract=Range of bits  numBits=8  bitIdxRange=[3 4]  outScalingMode=Preserve fixed-point scaling
      settings: SourceProductName=Simulink
  Extract Bits3 : simulink/Logic and Bit Operations/Extract Bits  bitsToExtract=Range of bits  numBits=8  bitIdxRange=[5 6]  outScalingMode=Preserve fixed-point scaling
      settings: SourceProductName=Simulink
  Extract Bits4 : simulink/Logic and Bit Operations/Extract Bits  bitsToExtract=Range of bits  numBits=8  bitIdxRange=7  outScalingMode=Preserve fixed-point scaling
      settings: SourceProductName=Simulink
  Gain : Gain  Gain=2^-0
  Gain1 : Gain  Gain=2^-8
  Gain2 : Gain  Gain=2^-3
  Gain3 : Gain  Gain=2^-5
  Gain4 : Gain  Gain=2^-7
  Licht_Auto : Outport
  Licht_TFL : Outport  Port=2
  Licht_ABL : Outport  Port=3
  Licht_FEL : Outport  Port=4
  Blinker_R_Tipp : Outport  Port=5
  Blinker_R : Outport  Port=6
  Blinker_L_Tipp : Outport  Port=7
  Blinker_L : Outport  Port=8
  Warnblinker : Outport  Port=9
  Licht_RFL : Outport  Port=10
  Trigger : Outport  Port=11
  wires:
  Extract Bits2/1 -> Gain2/1
  CanData_Cockpit_1/1 -> Extract Bits1/1, Extract Bits4/1, Extract Bits3/1, Extract Bits2/1, Extract Bits/1
  Extract Bits3/1 -> Gain3/1
  Gain/1 -> Compare To Constant3/1, Compare To Constant2/1, Compare To Constant1/1, Compare To Constant/1
  Gain3/1 -> Compare To Constant7/1, Compare To Constant6/1
  Compare To Constant3/1 -> Licht_FEL/1
  Gain1/1 -> Compare To Constant4/1
  Compare To Constant4/1 -> Licht_RFL/1
  Compare To Constant7/1 -> Detect Change3/1, Blinker_L/1
  Gain2/1 -> Compare To Constant9/1, Compare To Constant8/1
  Compare To Constant1/1 -> Licht_TFL/1
  Compare To Constant6/1 -> Detect Change2/1, Blinker_L_Tipp/1
  Compare To Constant5/1 -> Detect Change4/1, Warnblinker/1
  Compare To Constant8/1 -> Detect Change/1, Blinker_R_Tipp/1
  Compare To Constant/1 -> Licht_Auto/1
  Compare To Constant2/1 -> Licht_ABL/1
  Compare To Constant9/1 -> Detect Change1/1, Blinker_R/1
  Gain4/1 -> Compare To Constant5/1
  Extract Bits4/1 -> Gain4/1
  Extract Bits/1 -> Gain/1
  Extract Bits1/1 -> Gain1/1
  Detect Change/1 -> Bitwise Operator3/1
  Detect Change1/1 -> Bitwise Operator3/2
  Detect Change2/1 -> Bitwise Operator3/3
  Detect Change3/1 -> Bitwise Operator3/4
  Detect Change4/1 -> Bitwise Operator3/5
  Bitwise Operator3/1 -> Trigger/1

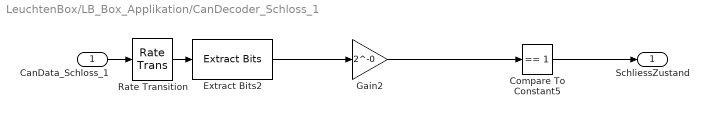
== system LeuchtenBox/LB_Box_Applikation/CanDecoder_Schloss_1 ==
  CanData_Schloss_1 : Inport
  Compare To Constant5 : simulink/Logic and Bit Operations/Compare To Constant  relop===  const=1  OutDataTypeStr=boolean
  Extract Bits2 : simulink/Logic and Bit Operations/Extract Bits  bitsToExtract=Range of bits  numBits=8  bitIdxRange=0  outScalingMode=Preserve fixed-point scaling
  Gain2 : Gain  Gain=2^-0
  Rate Transition : RateTransition  Deterministic=off
  SchliessZustand : Outport
  wires:
  Gain2/1 -> Compare To Constant5/1
  Extract Bits2/1 -> Gain2/1
  Compare To Constant5/1 -> SchliessZustand/1
  CanData_Schloss_1/1 -> Rate Transition/1
  Rate Transition/1 -> Extract Bits2/1

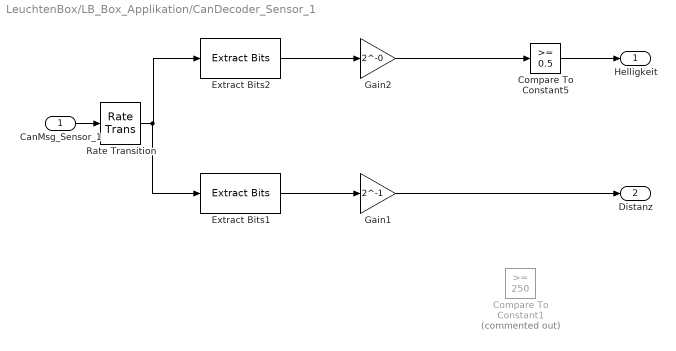
== system LeuchtenBox/LB_Box_Applikation/CanDecoder_Sensor_1 ==
  CanMsg_Sensor_1 : Inport
  Compare To Constant1 : simulink/Logic and Bit Operations/Compare To Constant  Commented=on  relop=>=  const=250  OutDataTypeStr=boolean
  Compare To Constant5 : simulink/Logic and Bit Operations/Compare To Constant  relop=>=  const=0.5  OutDataTypeStr=boolean
  Extract Bits1 : simulink/Logic and Bit Operations/Extract Bits  bitsToExtract=Range of bits  numBits=8  bitIdxRange=[1 9]  outScalingMode=Preserve fixed-point scaling
  Extract Bits2 : simulink/Logic and Bit Operations/Extract Bits  bitsToExtract=Range of bits  numBits=8  bitIdxRange=0  outScalingMode=Preserve fixed-point scaling
  Gain1 : Gain  Gain=2^-1
  Gain2 : Gain  Gain=2^-0
  Rate Transition : RateTransition  Deterministic=off
  Helligkeit : Outport
  Distanz : Outport  Port=2
  wires:
  Compare To Constant5/1 -> Helligkeit/1
  Extract Bits2/1 -> Gain2/1
  Gain2/1 -> Compare To Constant5/1
  Extract Bits1/1 -> Gain1/1
  CanMsg_Sensor_1/1 -> Rate Transition/1
  Rate Transition/1 -> Extract Bits1/1, Extract Bits2/1
  Gain1/1 -> Distanz/1

== stateflow chart LeuchtenBox/LB_Box_Applikation/Steuerung_Blinker ==
  state Blinken_AUS [parallel] [commented out]
    entry:
    BLL_LED=false;
    BLR_LED=false;
    L_needed=false;
    R_needed=false;
    freq_in_Hz=0;
    blink_count=0;
    StatusWB=false;
  state Blinken_EIN [parallel] [commented out]
    state Blinker_L [parallel] [commented out]
      state UNNEEDED [commented out]
      state NEEDED [commented out]
        during:
        BLL_LED=Takt;
      (default) -> Blinken_EIN.Blinker_L.UNNEEDED [commented out]
      Blinken_EIN.Blinker_L.UNNEEDED -> Blinken_EIN.Blinker_L.NEEDED [commented out] : [L_needed==true]
      Blinken_EIN.Blinker_L.NEEDED -> Blinken_EIN.Blinker_L.UNNEEDED [commented out] : [L_needed==false]
    state Blinker_R [parallel] [commented out]
      state UNNEEDED [commented out]
      state NEEDED [commented out]
        during:
        BLR_LED=Takt;
      (default) -> Blinken_EIN.Blinker_R.UNNEEDED [commented out]
      Blinken_EIN.Blinker_R.UNNEEDED -> Blinken_EIN.Blinker_R.NEEDED [commented out] : [R_needed==true]
      Blinken_EIN.Blinker_R.NEEDED -> Blinken_EIN.Blinker_R.UNNEEDED [commented out] : [R_needed==false]
    state Taktgeber [parallel] [commented out]
      state HIGH [commented out]
        entry:
        Takt=true;
      state LOW [commented out]
        entry:
        Takt=false;
        blink_count=blink_count-1;
      (default) -> Blinken_EIN.Taktgeber.HIGH [commented out]
      Blinken_EIN.Taktgeber.HIGH -> Blinken_EIN.Taktgeber.LOW [commented out] : after(1/freq_in_Hz, sec)
      Blinken_EIN.Taktgeber.LOW -> Blinken_EIN.Taktgeber.HIGH [commented out] : after(1/freq_in_Hz, sec)
  state Tippunterbrechung [parallel] [commented out]
  state STEUERUNG_RL [parallel]
    settings: executionOrder=1
    state AN
      entry:
      Blinken_R=false;
      Blinken_L=false;
      Warnblinken=false;
    state WARNBLINKEN
      during:
      Blinken_R=true;
      Blinken_L=true;
      freq_in_Hz=2;
      Warnblinken=true;
    state SCHLIESSBLINKEN
      entry:
      Blinken_R=true;
      Blinken_L=true;
      freq_in_Hz=2;
      blink_count=0;
    state warten
      entry:
      Blinken_R=false;
      Blinken_L=false;
    state OFFENBLINKEN
      entry:
      Blinken_R=true;
      Blinken_L=true;
      freq_in_Hz=2;
      blink_count=0;
    state ALARMBLINKEN
      during:
      Blinken_R=true;
      Blinken_L=true;
      freq_in_Hz=1;
    (default) -> STEUERUNG_RL.AN
    STEUERUNG_RL.AN -> STEUERUNG_RL.WARNBLINKEN [order 1] : [Warnblinker==true]
    STEUERUNG_RL.WARNBLINKEN -> STEUERUNG_RL.AN : [Warnblinker==false]
    STEUERUNG_RL.AN -> SCHLIESSBLINKEN [order 2] : [SchliessZustandTriggered==1 && SchliessZustand == 1]
    SCHLIESSBLINKEN -> STEUERUNG_RL.AN [order 2] : [Warnblinker==true]
    SCHLIESSBLINKEN -> warten [order 1] : [blink_count==2]
    warten -> STEUERUNG_RL.AN [order 3] : [Warnblinker==true]
    warten -> ALARMBLINKEN [order 2] : [AlarmZustand==1]
    warten -> OFFENBLINKEN [order 1] : [SchliessZustand == 0]
    STEUERUNG_RL.AN -> OFFENBLINKEN [order 3] : [SchliessZustandTriggered==1 && SchliessZustand==0]
    OFFENBLINKEN -> STEUERUNG_RL.AN : [blink_count==1 || Warnblinker==true]
    ALARMBLINKEN -> STEUERUNG_RL.AN [order 1] : [AlarmZustand==0]
    STEUERUNG_RL.AN -> ALARMBLINKEN [commented out] : [AlarmZustand==1]
    ALARMBLINKEN -> STEUERUNG_RL.AN [order 2] : [Warnblinker==true]
  state STEUERUNG_R [parallel]
    settings: executionOrder=2
    state AN
      entry:
      Blinken_R=false;
    state RECHTS
      entry:
      Blinken_R=true;
      freq_in_Hz=2;
    state WARNBLINKEN
    state FERTIG
      en, du: Blinken_R=true;
    state RECHTS_TIP
      entry:
      blink_count=0;
      during:
      Blinken_R=true;
      freq_in_Hz=2;
    (default) -> STEUERUNG_R.AN
    RECHTS -> STEUERUNG_R.AN [order 1] : [Blinker_R==0]
    STEUERUNG_R.AN -> RECHTS [order 1] : [Blinker_R==1]
    RECHTS -> STEUERUNG_R.WARNBLINKEN [order 2] : [Warnblinken==true]
    STEUERUNG_R.AN -> STEUERUNG_R.WARNBLINKEN [order 2] : [Warnblinken==true]
    STEUERUNG_R.WARNBLINKEN -> STEUERUNG_R.AN : [Warnblinken==false]
    STEUERUNG_R.AN -> RECHTS_TIP [order 3] : [Blinker_Tip_R==1]
    STEUERUNG_R.FERTIG -> STEUERUNG_R.AN : [Blinker_Tip_R==0]
    RECHTS_TIP -> STEUERUNG_R.WARNBLINKEN [order 2] : [Warnblinken==true]
    RECHTS_TIP -> STEUERUNG_R.FERTIG [order 3] : [Blinken_L==true]
    RECHTS_TIP -> STEUERUNG_R.FERTIG [order 1] : [blink_count==3]
  state BLINKER_RECHTS [parallel]
    settings: executionOrder=3
    state AUS
      entry:
      BLR_LED=false;
    state AN
      during:
      BLR_LED=Takt;
    (default) -> BLINKER_RECHTS.AUS
    BLINKER_RECHTS.AUS -> BLINKER_RECHTS.AN : [Blinken_R==true]
    BLINKER_RECHTS.AN -> BLINKER_RECHTS.AUS : [Blinken_R==false]
  state STEUERUNG_L [parallel]
    settings: executionOrder=6
    state AN
      entry:
      Blinken_L=false;
    state LINKS
      during:
      Blinken_L=true;
      freq_in_Hz=2;
    state WARNBLINKEN
    state FERTIG
      en, du: Blinken_L=true;
    state LINKS_TIP
      entry:
      blink_count=0;
      during:
      Blinken_L=true;
      freq_in_Hz=2;
    (default) -> STEUERUNG_L.AN
    LINKS -> STEUERUNG_L.AN [order 2] : [Blinker_L==0]
    STEUERUNG_L.AN -> LINKS [order 1] : [Blinker_L==1]
    LINKS -> STEUERUNG_L.WARNBLINKEN [order 1] : [Warnblinken==true]
    STEUERUNG_L.AN -> STEUERUNG_L.WARNBLINKEN [order 2] : [Warnblinken==true]
    STEUERUNG_L.WARNBLINKEN -> STEUERUNG_L.AN : [Warnblinken==false]
    LINKS_TIP -> STEUERUNG_L.WARNBLINKEN [order 3] : [Warnblinken==true]
    STEUERUNG_L.AN -> LINKS_TIP [order 3] : [Blinker_Tip_L==1]
    STEUERUNG_L.FERTIG -> STEUERUNG_L.AN : [Blinker_Tip_L==0]
    LINKS_TIP -> STEUERUNG_L.FERTIG [order 1] : [Blinken_R==true]
    LINKS_TIP -> STEUERUNG_L.FERTIG [order 2] : [blink_count==3]
  state BLINKER_LINKS [parallel]
    settings: executionOrder=5
    state AUS
      entry:
      BLL_LED=false;
    state AN
      during:
      BLL_LED=Takt;
    (default) -> BLINKER_LINKS.AUS
    BLINKER_LINKS.AUS -> BLINKER_LINKS.AN : [Blinken_L==true]
    BLINKER_LINKS.AN -> BLINKER_LINKS.AUS : [Blinken_L==false]
  state Taktgeber [parallel]
    entry:
    blink_count=0;
    freq_in_Hz=1;
    settings: executionOrder=4
    state HIGH
      entry:
      Takt=true;
    state Alarm
    state Alarm1
    state LOW
      entry:
      Takt=false;
      blink_count=blink_count+1;
    (default) -> Taktgeber.HIGH
    Taktgeber.HIGH -> Taktgeber.LOW [order 2] : after(0.25, sec)
    Taktgeber.LOW -> Taktgeber.HIGH [order 2] : after(0.25, sec)
    Alarm -> Taktgeber.HIGH : after(0.5, sec)
    Taktgeber.HIGH -> Alarm1 [order 1] : [AlarmZustand==1]
    Taktgeber.LOW -> Alarm [order 1] : [AlarmZustand==1]
    Alarm1 -> Taktgeber.LOW : after(0.5, sec)
  (default) -> Blinken_AUS [commented out] : {vorherigerSZ=2}
  Blinken_AUS -> Blinken_EIN [commented out] : [Blinker_L==1]{L_needed=true; freq_in_Hz=2}
  Blinken_AUS -> Blinken_EIN [commented out] : [Blinker_R==1]{R_needed=true; freq_in_Hz=2}
  Blinken_AUS -> Blinken_EIN [commented out] : [Blinker_Tip_L==1]{L_needed=true; freq_in_Hz=2; blink_count=3}
  Blinken_AUS -> Blinken_EIN [commented out] : [Blinker_Tip_R==1]{R_needed=true; freq_in_Hz=2; blink_count=3}
  Blinken_AUS -> Blinken_EIN [commented out] : [SchliessZustand==1 && (vorherigerSZ==0 || vorherigerSZ==2)]{L_needed=true; R_needed=true; freq_in_Hz=2; blink_count=2; vorherigerSZ=1}
  Blinken_AUS -> Blinken_EIN [commented out] : [SchliessZustand==0 && (vorherigerSZ==1)]{L_needed=true; R_needed=true; freq_in_Hz=2; blink_count=1; vorherigerSZ=0}
  Blinken_AUS -> Blinken_EIN [commented out] : [AlarmZustand==1]{L_needed=true; R_needed=true; freq_in_Hz=1}
  Blinken_AUS -> (junction 340) [commented out] : [Warnblinker==1 && StatusWB==false]
  (junction 340) -> Blinken_EIN [commented out] : {L_needed=true; R_needed=true; freq_in_Hz=2; StatusWB=true}
  Blinken_EIN -> (junction 340) [commented out] : [Warnblinker==1 && StatusWB==false]
  Blinken_EIN -> Blinken_AUS [commented out] : [Blinker_L==1 && Blinker_Tip_R==1]
  Blinken_EIN -> Blinken_AUS [commented out] : [Blinker_R==1 && Blinker_Tip_L==1]
  Blinken_EIN -> Blinken_AUS [commented out] : [Blinker_L==0 && Blinker_R==0 && blink_count==0 && Warnblinker==0 && AlarmZustand==0]
  Blinken_EIN -> Tippunterbrechung [commented out] : [(Blinker_Tip_L==1 || Blinker_Tip_R==1) && blink_count==0]
  Tippunterbrechung -> Blinken_AUS [commented out] : [(Blinker_Tip_L==0 && Blinker_Tip_R==0) || Warnblinker==1]
  data: BLL_LED output boolean; BLR_LED output boolean; Blinker_Tip_R input; Blinker_R input; Blinker_Tip_L input; Blinker_L input; Warnblinker input boolean; SchliessZustand input boolean; AlarmZustand input; Count local; OpeningCount local; ClosingCount local; Opening local; Closing local; blink_left local boolean; blink_right local boolean; blink_count local uint32; blink_delay local double; SchliessZustandTriggered input; AlarmZustandTriggered input; WarnBremse input; NotBremse input; Takt local boolean; L_needed local boolean; R_needed local boolean; vorherigerSZ local int8; StatusWB local boolean; Blinken_R_TIP local boolean; Blinken_R local boolean; Warnblinken local boolean; Blinken_L_TIP local boolean; Blinken_L local boolean; freq_in_Hz local int8; message output; Trigger input
  events: SchliessZustandUpdated local FUNCTION_CALL_EVENT; AlarmZustandUpdated local FUNCTION_CALL_EVENT

== stateflow chart LeuchtenBox/LB_Box_Applikation/Steuerung_Bremslicht ==
  state Bremslicht
    during:
    BL_LED=Bremse;
  (default) -> Bremslicht
  data: BL_LED output boolean; Bremse input boolean; WarnBremse input boolean; NotBremse input boolean

== stateflow chart LeuchtenBox/LB_Box_Applikation/Steuerung_Licht2 ==
  state Lichtsteuerung [parallel]
    settings: executionOrder=1
    state Schalter_AUS
      entry:
      FEL_LED=false;
      ABL_LED=false;
      TFL_LED=false;
      RL_LED=false;
      KLL_LED=false;
      KLR_LED=false;
    state Schalter_MANUELL
      state Schalterstellung
      state Stufe_0_TFL
        entry:
        TFL_LED=true;
        ABL_LED=false;
        FEL_LED=false;
        RL_LED=false;
      state Stufe_1_ABL
        entry:
        TFL_LED=false;
        ABL_LED=true;
        FEL_LED=false;
        RL_LED=true;
      state Stufe_2_FEL
        entry:
        TFL_LED=false;
        ABL_LED=false;
        FEL_LED=true;
        RL_LED=true;
      (default) -> Schalterstellung
      Schalterstellung -> Stufe_0_TFL [order 1] : [Licht_TFL==1]
      Stufe_0_TFL -> Schalterstellung : [Licht_TFL==0]
      Schalterstellung -> Stufe_1_ABL [order 2] : [Licht_ABL==1]
      Stufe_1_ABL -> Schalterstellung : [Licht_ABL==0]
      Schalterstellung -> Stufe_2_FEL [order 3] : [Licht_FEL==1]
      Stufe_2_FEL -> Schalterstellung : [Licht_FEL==0]
    state Schalter_AUTO
      state DUNKEL
        state GEGENVERKEHR
          entry:
          TFL_LED=false;
          ABL_LED=true;
          FEL_LED=false;
          RL_LED=true;
        state KEIN_GEGENVERKEHR
          entry:
          TFL_LED=false;
          ABL_LED=false;
          FEL_LED=true;
          RL_LED=true;
        (default) -> GEGENVERKEHR
        GEGENVERKEHR -> KEIN_GEGENVERKEHR : [Distanz>=250]
        KEIN_GEGENVERKEHR -> GEGENVERKEHR : [Distanz<250]
      state HELL
        entry:
        TFL_LED=true;
        ABL_LED=false;
        FEL_LED=false;
        RL_LED=false;
      (default) -> DUNKEL
      DUNKEL -> HELL : [Helligkeit==1]
      HELL -> DUNKEL : [Helligkeit==0]
    (default) -> Schalter_AUS
    Schalter_AUS -> Schalter_AUTO [order 2] : [Licht_Auto==1]
    Schalter_AUTO -> Schalter_AUS [order 1] : [Licht_TFL==0 && Licht_ABL==0 && Licht_FEL==0 && Licht_Auto==0]
    Schalter_AUS -> Schalter_MANUELL [order 1] : [Licht_TFL==1 || Licht_ABL==1 || Licht_FEL==1]
    Schalter_MANUELL -> Schalter_AUS [order 1] : [Licht_TFL==0 && Licht_ABL==0 && Licht_FEL==0 && Licht_Auto==0]
    Schalter_MANUELL -> Schalter_AUTO [order 2] : [Licht_Auto==1]
    Schalter_AUTO -> Schalter_MANUELL [order 2] : [Licht_TFL==1 || Licht_ABL==1 || Licht_FEL==1]
  state Rueckfahrlicht [parallel]
    settings: executionOrder=2
    state RFL_OFF
      entry:
      RFL_LED=false;
    state RFL_ON
      entry:
      RFL_LED=true;
    (default) -> RFL_OFF
    RFL_OFF -> RFL_ON : [Licht_RFL==1]
    RFL_ON -> RFL_OFF : [Licht_RFL==0 ]
  data: FEL_LED output boolean; Helligkeit input boolean; Distanz input; ABL_LED output boolean; TFL_LED output boolean; Licht_Auto input boolean; Licht_TFL input boolean; Licht_ABL input boolean; Licht_FEL input boolean; RL_LED output boolean; KLL_LED output boolean; KLR_LED output boolean; Licht_RFL input boolean; RFL_LED output boolean
